simulink model "dtm"  (R2023b)
settings: Solver=ode45  StartTime=0.0  StopTime=15  RelTol=1e-3  EnableMultiTasking=on
settings Model: Creator=eechris  LastModifiedBy=eechris
settings SolverCC: AlgebraicLoopSolver=TrustRegion
settings DataIOCC: LimitDataPoints=on  SaveFormat=Array  ReturnWorkspaceOutputs=off
settings OptimizationCC: ExpressionDepthLimit=2147483647  LifeSpan=inf
settings DebuggingCC: UnderspecifiedInitializationDetection=Classic  MergeDetectMultiDrivingBlocksExec=none  SolverPrmCheckMsg=warning  UnconnectedInputMsg=warning  UnconnectedOutputMsg=warning  UnconnectedLineMsg=warning  StateNameClashWarn=warning  SFUnexpectedBacktrackingDiag=warning  SFNoUnconditionalDefaultTransitionDiag=warning  SFExecutionAtInitializationDiag=none  ArithmeticOperatorsInVariantConditions=warning
settings HardwareCC: ProdBitPerPointer=32  ProdBitPerSizeT=32  ProdBitPerPtrDiffT=32  ProdLargestAtomicFloat=None  ProdIntDivRoundTo=Undefined  ProdEndianess=Unspecified  ProdWordSize=32  ProdHWDeviceType=32-bit Generic
settings ModelReferenceCC: PropagateSignalLabelsOutOfModel=off
settings SFSimCC: SimUseLocalCustomCode=off  CustomCodeUndefinedFunction=UseInterfaceOnly
settings RTWCC: RTWUseLocalCustomCode=off
settings CodeAppCC: StateflowObjectComments=on
settings GRTTargetCC: TargetLangStandard=C89/C90 (ANSI)
settings ConfigComp: CovMetricSettings=dw  CovSaveCumulativeToWorkspaceVar=on  CovSaveSingleToWorkspaceVar=on  CovExternalEMLEnable=off

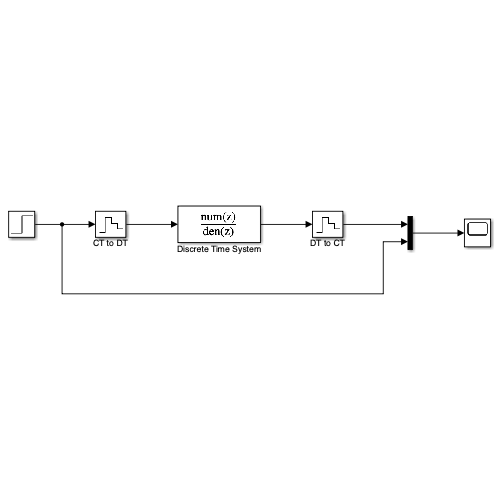
[thumbnail: Simulink's stored preview of the top-level diagram]
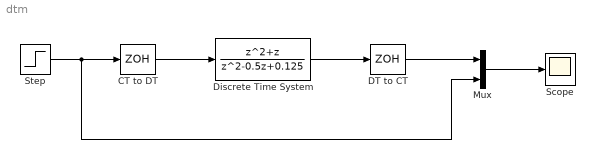
== system dtm ==
  CT to DT : ZeroOrderHold
  DT to CT : ZeroOrderHold
  Discrete Time System : DiscreteTransferFcn  Numerator=[1 1 0]  Denominator=[1 -0.5 0.125]
  Mux : Mux  Inputs=2
  Scope : Scope
  Step : Step  SampleTime=0
  wires:
  Step/1 -> Mux/2, CT to DT/1
  CT to DT/1 -> Discrete Time System/1
  Discrete Time System/1 -> DT to CT/1
  DT to CT/1 -> Mux/1
  Mux/1 -> Scope/1
